simulink model "dvbt_sim"  (Simulink 6.0)
settings: Solver=VariableStepDiscrete  SolverMode=SingleTasking  StartTime=0.0  StopTime=0.004  RelTol=1e-3
model workspace: external: M-Code (data not in the file)
values from neighbouring files (symbols this model uses):
  Ts = 2.857893354347255e-007    (= 2.85789335435e-07)    [dvbt_table_gen.m]
undefined symbols (not defined in the file or in its folder): EbNodB, figposition, Fs, M, rsgenpoly, slcm
libraries: commutil2 x5, commblkintrlv2 x4, dspbuff3 x4, commsink2 x3, commblkcod2 x2, simulink x2, commcnvcod2 x2, commsequence2 x2, dspsigops x2, dspxfrm3 x2, commcnvintrlv2 x2, commchan2 x1
CloseFcn:
  | % Clear global variables
  | clear global GF_TABLE1 GF_TABLE2 GF_TABLE_M GF_TABLE_PRIM_POLY
  | 
  | % Clear signal logging variable
  | clear dvbSigsOut
settings Model: Creator=mikem  LastModifiedBy=arodrigu  ExtModeTrigMode=oneshot  ExtModeArmWhenConnect=off  BufferReuse=off
settings SolverCC: ZeroCrossControl=DisableAll
settings DataIOCC: LimitDataPoints=off  SaveOutput=off  SaveTime=off  SignalLoggingName=dvbSigsOut
settings OptimizationCC: BlockReduction=off  BooleanDataType=off  InlineInvariantSignals=off  OptimizeBlockIOStorage=off  BufferReuse=off  ExpressionFolding=off  LocalBlockOutputs=off
settings DebuggingCC: CheckExecutionContextPreStartOutputMsg=on  CheckExecutionContextRuntimeOutputMsg=on  SolverPrmCheckMsg=none  InheritedTsInSrcMsg=none
settings HardwareCC: TargetHWDeviceType=MATLAB Host  ProdEqTarget=off
settings ModelReferenceCC: UpdateModelReferenceTargets=IfOutOfDate
settings RTWCC: SystemTargetFile=rsim.tlc  TemplateMakefile=rsim_default_tmf  ProcessScript=rsim_make_rtw_hook
settings RSimTargetCC: TargetFcnLib=ansi_tfl_tmw.mat  GenFloatMathFcnCalls=ANSI_C  IsPILTarget=off

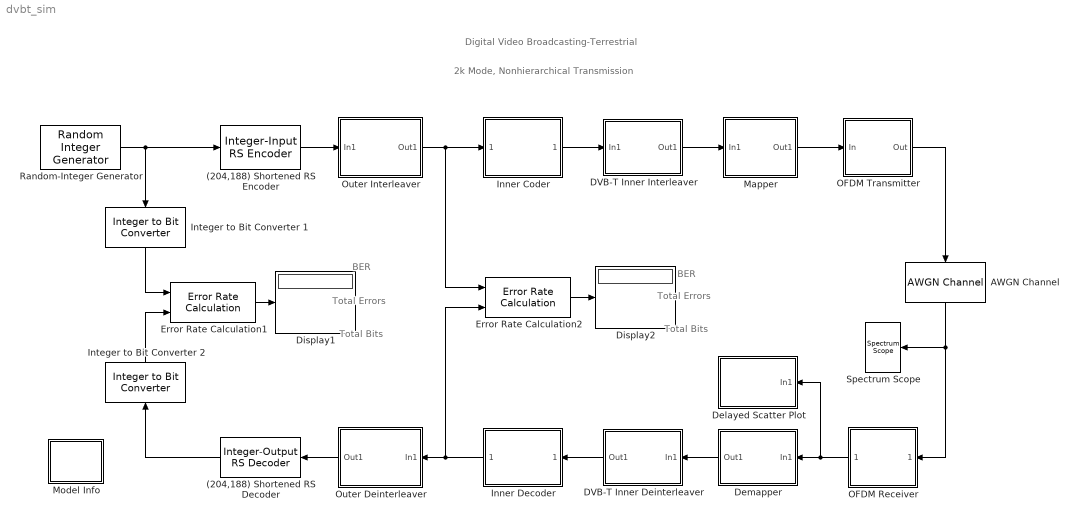
== system dvbt_sim ==
  note: Digital Video Broadcasting-Terrestrial
  note: 2k Mode, Nonhierarchical Transmission
  note: BER
  note: Total Errors
  note: Total Bits
  note: Total Errors
  note: Total Bits
  note: BER
  (204,188) Shortened RS Decoder : commblkcod2/Integer-Output RS Decoder  Orientation=left  n=204  k=188  specPrimPoly=off  primPoly=[1 0 1 1]  specGenPoly=off  genPoly=rsgenpoly(7,3)  showNumErr=off
  (204,188) Shortened RS Encoder : commblkcod2/Integer-Input RS Encoder  n=204  k=188  specPrimPoly=off  primPoly=[1 0 1 1]  specGenPoly=off  genPoly=rsgenpoly(7,3)
  AWGN Channel : commchan2/AWGN Channel  Orientation=down  seed=54321  noiseMode="Signal to noise ratio  (SNR)"  EbNodB=10  EsNodB=EbNodB+10*log10(log2(M))  SNRdB=18.5  bitsPerSym=1  Ps=1/2048  Tsym=Tsym  variance=10^(-0.1*15)/(2048*2)
  DVB-T Inner Deinterleaver : Subsystem  Orientation=left  PropExecContextAcrossSSBoundary=on  mask(DVB-T Inner Deinterleaver){}
      mask init:
      | fullILVec = [(1:126) ...
      |  (rem([0:125]+63,126) +1 + 126     ) ...
      |  (rem([0:125]+105,126)+1 + (2*126) ) ...
      |  (rem([0:125]+42,126) +1 + (3*126) ) ...
      |  (rem([0:125]+21,126) +1 + (4*126) ) ...
      |  (rem([0:125]+84,126) +1 + (5*126) )];
      mask Display: disp('DVB-T\nInner\nDeinterleaver')
  DVB-T Inner Interleaver : Subsystem  PropExecContextAcrossSSBoundary=on  mask(DVB-T Inner Interleaver){}
      mask init: same as dvbt_sim/DVB-T Inner Deinterleaver
      mask Display: disp('DVB-T\nInner\nInterleaver')
  Delayed Scatter Plot : Subsystem  Orientation=left  PropExecContextAcrossSSBoundary=on
      mask Display: disp('Delayed\nScatter Plot');
  Demapper : Subsystem  Orientation=left  PropExecContextAcrossSSBoundary=on
      mask Type: DVB-T 64-QAM Demapper
      mask Display: disp('DVB-T\n64-QAM\nDemapper')
  Display1 : Display
  Display2 : Display
  Error Rate Calculation1 : commsink2/Error Rate Calculation  N=188*17*8  st_delay=0  cp_mode=Entire frame  subframe=[]  PMode=Port  WsName=e2  RsMode2=off  stop=off  numErr=100  maxBits=1e6
  Error Rate Calculation2 : commsink2/Error Rate Calculation  N=1632*6  st_delay=0  cp_mode=Entire frame  subframe=[]  PMode=Port  WsName=e1  RsMode2=off  stop=off  numErr=100  maxBits=1e6
  Inner Coder : Subsystem  PropExecContextAcrossSSBoundary=on
      mask Display: disp('Rate 3/4\nPunctured\nConvolutional\nCode');
  Inner Decoder : Subsystem  Orientation=left  PropExecContextAcrossSSBoundary=on
      mask Display: disp('Viterbi\nDecoder')
  Integer to Bit Converter 1 : commutil2/Integer to Bit Converter  Orientation=down  nbits=8
  Integer to Bit Converter 2 : commutil2/Integer to Bit Converter  Orientation=up  nbits=8
  Mapper : Subsystem  PropExecContextAcrossSSBoundary=on
      mask Type: DVB-T 64-QAM Mapper
      mask Display: disp('DVB-T\n64-QAM\nMapper')
  Model Info : Subsystem  LoadFcn=slcm LoadBlock;  InitFcn=slcm('UpdateAllCMBlocksInThisModelInit')  PropExecContextAcrossSSBoundary=on  mask(CMBlock){InitialSaveTempField=, InitialBlockCM=none, BlockCM=none, Frame=on, SaveTempField=, DisplayStringWithTags=Info, MaskDisplayString=Info, HorizontalTextAlignment=Center, LeftAlignmentValue=0.5, SourceBlockDiagram=dvbt_sim, TagMaxNumber=20, CMTag1=, CMTag2=, CMTag3=, CMTag4=, CMTag5=, CMTag6=, CMTag7=, CMTag8=, CMTag9=, CMTag10=, CMTag11=, CMTag12=, CMTag13=, CMTag14=, CMTag15=, CMTag16=, CMTag17=, CMTag18=, CMTag19=, CMTag20=}
      mask help: This block allows revision control information to be displayed within the model.
      settings: CopyFcn=slcm CopyBlock;  DeleteFcn=slcm Cancel;  PostSaveFcn=slcm('UpdateAllCMBlocksInThisModel')  NameChangeFcn=slcm Rename;  OpenFcn=commdemohelp;
      mask Display: text(str2num(LeftAlignmentValue), 0.5, MaskDisplayString, 'HorizontalAlignment', HorizontalTextAlignment)
  OFDM Receiver : Subsystem  Orientation=left  PropExecContextAcrossSSBoundary=on
      mask Display: disp('OFDM\nReceiver')
  OFDM Transmitter : Subsystem  PropExecContextAcrossSSBoundary=on
      mask Display: disp('OFDM\nTransmitter')
  Outer Deinterleaver : Subsystem  Orientation=left  PropExecContextAcrossSSBoundary=on
      mask Type: Convolutional Deinterleaver
      mask Display: disp('Convolutional\nDeinterleaver\nI=12')
  Outer Interleaver : Subsystem  PropExecContextAcrossSSBoundary=on
      mask Type: Convolutional Interleaver
      mask Display: disp('Convolutional\nInterleaver\nI=12')
  Random-Integer Generator : commrandsrc2/Random Integer Generator  mul=256  seed=1234573  Ts=Ts  frameBased=on  sampPerFrame=188  orient=off
  Spectrum Scope : dspsnks4/Spectrum Scope  Orientation=left  ScopeProperties=off  Domain=Frequency  HorizSpan=1  UseBuffer=off  BufferSize=128  Overlap=64  inpFftLenInherit=off  FFTlength=128  numAvg=2  DisplayProperties=on  AxisGrid=on  Memory=off  FrameNumber=off  AxisLegend=off  AxisZoom=off  OpenScopeAtSimStart=on  OpenScopeImmediately=off  FigPos="figposition([9    38    30    30])"  AxisProperties=off  XUnits=Hertz  XRange=[-Fs/2...Fs/2]  InheritXIncr=on  XIncr=1.0  XLabel=Samples  YUnits=dB  YLabel=Magnitude, dB  LineProperties=off
      settings: YMin=-100  YMax=20
  wires:
  Random-Integer Generator/1 -> Integer to Bit Converter 1/1, (204,188) Shortened RS Encoder/1
  Mapper/1(Out1) -> OFDM Transmitter/1(In)
  (204,188) Shortened RS Encoder/1 -> Outer Interleaver/1(In1)
  Outer Interleaver/1(Out1) -> Error Rate Calculation2/1, Inner Coder/1(Uncoded symbols)
  OFDM Transmitter/1(Out) -> AWGN Channel/1
  OFDM Receiver/1(OFDM Spectrum) -> Demapper/1(In1), Delayed Scatter Plot/1(In1)
  DVB-T Inner Deinterleaver/1(Out1) -> Inner Decoder/1(Received bits)
  Inner Decoder/1(Decoded symbols) -> Outer Deinterleaver/1(In1), Error Rate Calculation2/2
  Outer Deinterleaver/1(Out1) -> (204,188) Shortened RS Decoder/1
  Error Rate Calculation1/1 -> Display1/1
  Error Rate Calculation2/1 -> Display2/1
  Integer to Bit Converter 2/1 -> Error Rate Calculation1/2
  Integer to Bit Converter 1/1 -> Error Rate Calculation1/1
  (204,188) Shortened RS Decoder/1 -> Integer to Bit Converter 2/1
  DVB-T Inner Interleaver/1(Out1) -> Mapper/1(In1)
  Inner Coder/1(Coded bits) -> DVB-T Inner Interleaver/1(In1)
  Demapper/1(Out1) -> DVB-T Inner Deinterleaver/1(In1)
  AWGN Channel/1 -> Spectrum Scope/1, OFDM Receiver/1(Received signal)

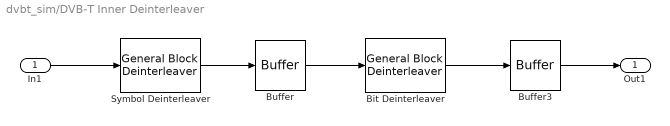
== system dvbt_sim/DVB-T Inner Deinterleaver ==
  In1 : Inport  LatchInput=off
  Bit Deinterleaver : commblkintrlv2/General Block Deinterleaver  elements=dvb_bit_int_table
  Buffer : dspbuff3/Buffer  N=756  V=0  ic=0
  Buffer3 : dspbuff3/Buffer  N=2176  V=0  ic=0
  Symbol Deinterleaver : commblkintrlv2/General Block Deinterleaver  elements=dvb_sym_int_table
  Out1 : Outport
  wires:
  Buffer/1 -> Bit Deinterleaver/1
  In1/1 -> Symbol Deinterleaver/1
  Bit Deinterleaver/1 -> Buffer3/1
  Buffer3/1 -> Out1/1
  Symbol Deinterleaver/1 -> Buffer/1

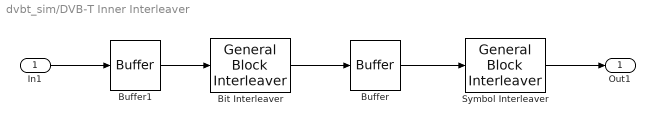
== system dvbt_sim/DVB-T Inner Interleaver ==
  In1 : Inport  LatchInput=off
  Bit Interleaver : commblkintrlv2/General Block Interleaver  elements=dvb_bit_int_table
  Buffer : dspbuff3/Buffer  N=9072  V=0  ic=0
  Buffer1 : dspbuff3/Buffer  N=756  V=0  ic=0
  Symbol Interleaver : commblkintrlv2/General Block Interleaver  elements=dvb_sym_int_table
  Out1 : Outport
  wires:
  Buffer1/1 -> Bit Interleaver/1
  In1/1 -> Buffer1/1
  Bit Interleaver/1 -> Buffer/1
  Symbol Interleaver/1 -> Out1/1
  Buffer/1 -> Symbol Interleaver/1

== system dvbt_sim/Delayed Scatter Plot ==
  In1 : Inport  LatchInput=off
  Enabled Scatter Plot : Subsystem  TreatAsAtomicUnit=on  PropExecContextAcrossSSBoundary=on
  Step : Step  Time=.001  SampleTime=.000224
  wires:
  Step/1 -> Enabled Scatter Plot/Enable
  In1/1 -> Enabled Scatter Plot/1(In1)

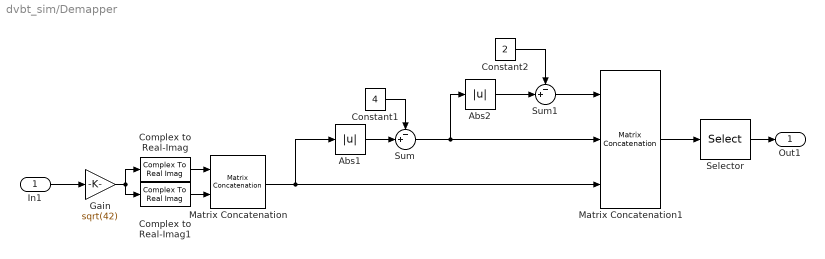
== system dvbt_sim/Demapper ==
  In1 : Inport  LatchInput=off
  Abs1 : Abs  SaturateOnIntegerOverflow=on
  Abs2 : Abs  SaturateOnIntegerOverflow=on
  Complex to Real-Imag : ComplexToRealImag  Output=Imag
  Complex to Real-Imag1 : ComplexToRealImag  Output=Real
  Constant1 : Constant  Value=4
  Constant2 : Constant  Value=2
  Gain : Gain  Gain=sqrt(42)  SaturateOnIntegerOverflow=on
  Matrix Concatenation : simulink/Math Operations/Matrix Concatenation  numInports=2  catMethod=Vertical
  Matrix Concatenation1 : simulink/Math Operations/Matrix Concatenation  numInports=3  catMethod=Vertical
  Selector : Selector  Elements=reshape(reshape(1:9072,1512,6)',9072,1)  InputPortWidth=9072
  Sum : Sum  Inputs=-+|  SaturateOnIntegerOverflow=on  InputSameDT=on
  Sum1 : Sum  Inputs=-+|  SaturateOnIntegerOverflow=on  InputSameDT=on
  Out1 : Outport
  wires:
  Matrix Concatenation/1 -> Abs1/1, Matrix Concatenation1/3
  Gain/1 -> Complex to Real-Imag/1, Complex to Real-Imag1/1
  Complex to Real-Imag1/1 -> Matrix Concatenation/2
  Complex to Real-Imag/1 -> Matrix Concatenation/1
  Sum/1 -> Abs2/1, Matrix Concatenation1/2
  Abs1/1 -> Sum/2
  Constant1/1 -> Sum/1
  Constant2/1 -> Sum1/1
  Abs2/1 -> Sum1/2
  Selector/1 -> Out1/1
  Sum1/1 -> Matrix Concatenation1/1
  In1/1 -> Gain/1
  Matrix Concatenation1/1 -> Selector/1

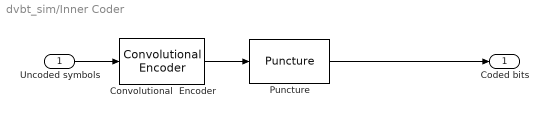
== system dvbt_sim/Inner Coder ==
  Uncoded symbols : Inport  LatchInput=off
  Convolutional  Encoder : commcnvcod2/Convolutional Encoder  trellis=poly2trellis(7, [171 133])  reset=None
  Puncture : commsequence2/Puncture  punctureVector=[1 1 0 1 1 0]'
  Coded bits : Outport
  wires:
  Convolutional  Encoder/1 -> Puncture/1
  Uncoded symbols/1 -> Convolutional  Encoder/1
  Puncture/1 -> Coded bits/1

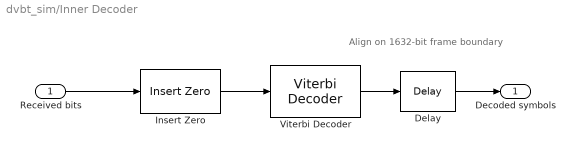
== system dvbt_sim/Inner Decoder ==
  note: Align on 1632-bit
      | frame boundary
  Received bits : Inport  LatchInput=off
  Delay : dspsigops/Delay  dly_unit=Samples  delay=584+69  ic_detail=off  dif_ic_for_ch=off  dif_ic_for_dly=off  ic=0  reset_popup=None
  Insert Zero : commsequence2/Insert Zero  insertZeroVector=[1 1 0 1 1 0]'
  Viterbi Decoder : commcnvcod2/Viterbi Decoder  trellis=poly2trellis(7, [171 133])  dectype=Unquantized  nsdecb=4  tbdepth=136  opmode=Continuous  reset=off
  Decoded symbols : Outport
  wires:
  Viterbi Decoder/1 -> Delay/1
  Insert Zero/1 -> Viterbi Decoder/1
  Received bits/1 -> Insert Zero/1
  Delay/1 -> Decoded symbols/1

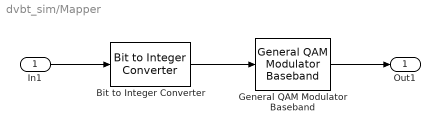
== system dvbt_sim/Mapper ==
  In1 : Inport  LatchInput=off
  Bit to Integer Converter : commutil2/Bit to Integer Converter  nbits=6
  General QAM Modulator Baseband : commdigbbndam2/General QAM Modulator Baseband  SigCon=dvbt_qam  numSamp=1
  Out1 : Outport
  wires:
  General QAM Modulator Baseband/1 -> Out1/1
  In1/1 -> Bit to Integer Converter/1
  Bit to Integer Converter/1 -> General QAM Modulator Baseband/1

== system dvbt_sim/Model Info ==
  EmptySubsystem : Subsystem  PropExecContextAcrossSSBoundary=on

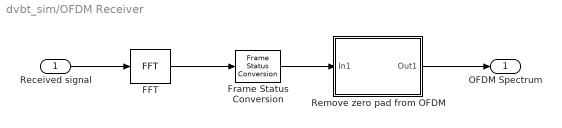
== system dvbt_sim/OFDM Receiver ==
  Received signal : Inport  LatchInput=off
  FFT : dspxfrm3/FFT  CompMethod=Table lookup  TableOpt=Speed  BitRevOrder=off  SkipNorm=off  firstCoeffMode=User-defined  firstCoeffWordLength=16  firstCoeffFracLength=15  roundingMode=Floor  overflowMode=off
  Frame Status Conversion : dspsigattribs/Frame Status Conversion  growRefPort=off  outframe=Frame-based
  Remove zero pad from OFDM : Subsystem  PropExecContextAcrossSSBoundary=on
      mask Display: disp('Remove zero\npad from OFDM');
  OFDM Spectrum : Outport
  wires:
  Remove zero pad from OFDM/1(Out1) -> OFDM Spectrum/1
  Received signal/1 -> FFT/1
  FFT/1 -> Frame Status Conversion/1
  Frame Status Conversion/1 -> Remove zero pad from OFDM/1(In1)

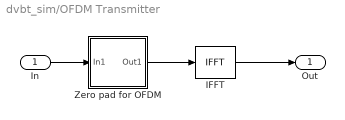
== system dvbt_sim/OFDM Transmitter ==
  In : Inport  LatchInput=off
  IFFT : dspxfrm3/IFFT  CompMethod=Table lookup  TableOpt=Speed  BitRevOrder=off  cs_in=off  SkipNorm=off  mode=Complex  firstCoeffMode=User-defined  firstCoeffWordLength=16  firstCoeffFracLength=15  roundingMode=Floor  overflowMode=off
  Zero pad for OFDM : Subsystem  PropExecContextAcrossSSBoundary=on
      mask Display: disp('Zero pad\nfor OFDM');
  Out : Outport
  wires:
  IFFT/1 -> Out/1
  In/1 -> Zero pad for OFDM/1(In1)
  Zero pad for OFDM/1(Out1) -> IFFT/1

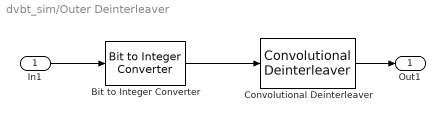
== system dvbt_sim/Outer Deinterleaver ==
  In1 : Inport  LatchInput=off
  Bit to Integer Converter : commutil2/Bit to Integer Converter  nbits=8
  Convolutional Deinterleaver : commcnvintrlv2/Convolutional Deinterleaver  N=12  B=17  ic=0
  Out1 : Outport
  wires:
  In1/1 -> Bit to Integer Converter/1
  Convolutional Deinterleaver/1 -> Out1/1
  Bit to Integer Converter/1 -> Convolutional Deinterleaver/1

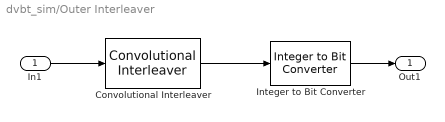
== system dvbt_sim/Outer Interleaver ==
  In1 : Inport  LatchInput=off
  Convolutional Interleaver : commcnvintrlv2/Convolutional Interleaver  N=12  B=17  ic=0
  Integer to Bit Converter : commutil2/Integer to Bit Converter  nbits=8
  Out1 : Outport
  wires:
  Integer to Bit Converter/1 -> Out1/1
  Convolutional Interleaver/1 -> Integer to Bit Converter/1
  In1/1 -> Convolutional Interleaver/1

== system dvbt_sim/Delayed Scatter Plot/Enabled Scatter Plot ==
  In1 : Inport  LatchInput=off
  Enable : EnablePort
  Discrete-Time Scatter Plot Scope : commsink2/Discrete-Time Scatter Plot Scope  Tag=ScatterPlot  sampPerSymb=1  offsetEye=0  numTraces=5000  numNewFrames=3000  LineMarkers=.  LineColors=b  fading=off  render=off  AxisGrid=on  xMin=-1.5  xMax=1.5  yMin=-1.5  yMax=1.5  inphaseLabel=In-phase Amplitude  quadratureLabel=Quadrature Amplitude  openScopeAtSimStart=on  FrameNumber=off  FigPos="figposition([50    18    44    58])"  figTitle=Scatter Plot  numLinesMax=50  block_type_=scatter
  wires:
  In1/1 -> Discrete-Time Scatter Plot Scope/1

== system dvbt_sim/Model Info/EmptySubsystem ==

== system dvbt_sim/OFDM Receiver/Remove zero pad from OFDM ==
  In1 : Inport  LatchInput=off
  Selector : Selector  Elements=[1:756 1293:2048]  InputPortWidth=2048
  Out1 : Outport
  wires:
  In1/1 -> Selector/1
  Selector/1 -> Out1/1

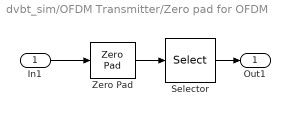
== system dvbt_sim/OFDM Transmitter/Zero pad for OFDM ==
  In1 : Inport  LatchInput=off
  Selector : Selector  Elements="[1:756 1513:2048  757:1512]"  InputPortWidth=2048
  Zero Pad : dspsigops/Zero Pad  padSigAt=End  zpadAlong=Columns  padNumOutRowsSpecMethod=User-specified  numOutRows=2048  padNumOutColsSpecMethod=User-specified  numOutCols=1  trunc_flag=None
  Out1 : Outport
  wires:
  In1/1 -> Zero Pad/1
  Selector/1 -> Out1/1
  Zero Pad/1 -> Selector/1
